simulink model "LAB7_OLD"  (R2021b)
settings: Solver=VariableStepDiscrete  StartTime=0.0  StopTime=100000  RelTol=1e-3  EnableMultiTasking=on
libraries: commchan3 x8, commdigbbndpm3 x8, commsink2 x8, commdigbbndam3 x8, commblkcod2 x8, commrandsrc3 x4
settings Model: Creator=The MathWorks, Inc.  LastModifiedBy=Argot
settings SolverCC: AlgebraicLoopSolver=TrustRegion
settings DataIOCC: LimitDataPoints=on  SaveFormat=Array  ReturnWorkspaceOutputs=off  SignalLoggingName=sigsOut
settings OptimizationCC: ExpressionDepthLimit=2147483647  InitFltsAndDblsToZero=on  LifeSpan=inf
settings DebuggingCC: SaveWithParameterizedLinksMsg=none  UnderspecifiedInitializationDetection=Classic  MergeDetectMultiDrivingBlocksExec=none  SignalResolutionControl=TryResolveAllWithWarning  MultiTaskDSMMsg=warning  MultiTaskCondExecSysMsg=none  FcnCallInpInsideContextMsg=warning  StateNameClashWarn=warning  SFUnexpectedBacktrackingDiag=warning  SFNoUnconditionalDefaultTransitionDiag=warning  SFExecutionAtInitializationDiag=none  SFMachineParentedDataDiag=warning  ArithmeticOperatorsInVariantConditions=warning
settings HardwareCC: ProdBitPerPointer=32  ProdBitPerSizeT=32  ProdBitPerPtrDiffT=32  ProdLargestAtomicFloat=None  ProdIntDivRoundTo=Undefined  ProdEndianess=Unspecified  ProdWordSize=32  ProdHWDeviceType=32-bit Generic  TargetUnknown=on
settings ModelReferenceCC: PropagateSignalLabelsOutOfModel=off
settings SFSimCC: SimUseLocalCustomCode=off  CustomCodeUndefinedFunction=UseInterfaceOnly
settings RTWCC: RTWUseLocalCustomCode=off
settings CodeAppCC: StateflowObjectComments=on
settings GRTTargetCC: TargetFcnLib=ansi_tfl_tmw.mat  TargetLangStandard=C89/C90 (ANSI)  CombineOutputUpdateFcns=off  GRTInterface=on
settings ConfigComp: CovMetricSettings=dw  CovSaveCumulativeToWorkspaceVar=on  CovSaveSingleToWorkspaceVar=on  CovExternalEMLEnable=off

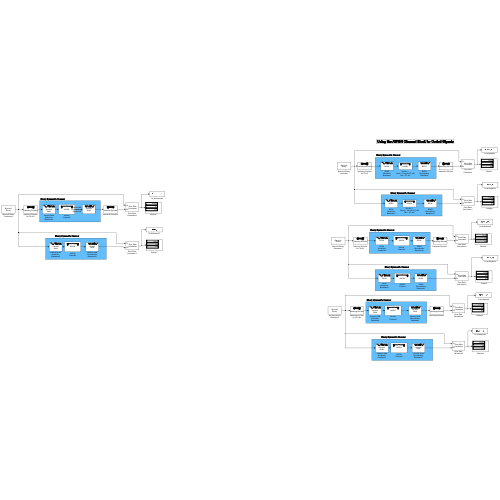
[thumbnail: Simulink's stored preview of the top-level diagram]
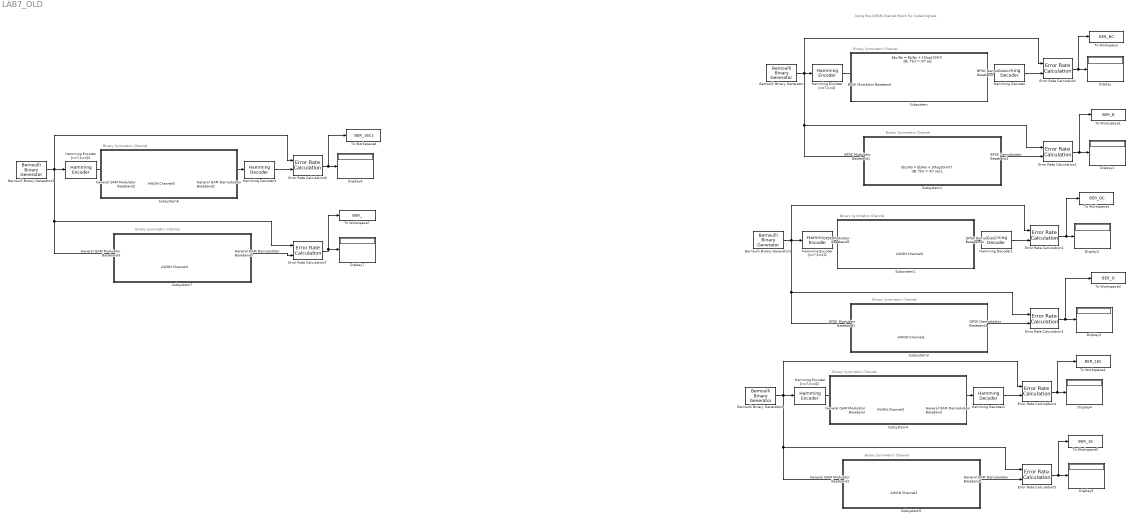
== system LAB7_OLD ==
  note: Binary Symmetric Channel
  note: Using the AWGN Channel Block for Coded Signals
  note: Binary Symmetric Channel
  note: Binary Symmetric Channel
  note: Binary Symmetric Channel
  note: Binary Symmetric Channel
  note: Binary Symmetric Channel
  note: Binary Symmetric Channel
  note: Binary Symmetric Channel
  AWGN Channel{1..3,6} (4 alike) : commchan3/AWGN Channel  InputProcessing=Columns as channels (frame based)  seed=67  noiseMode="Signal to noise ratio  (Eb/No)"  EbNodB=-40  EsNodB=10  SNRdB=10  bitsPerSym=1  Ps=1  Tsym=1  variance=1
  AWGN Channel4 : commchan3/AWGN Channel  InputProcessing=Columns as channels (frame based)  seed=67  noiseMode="Signal to noise ratio  (Eb/No)"  EbNodB=-2  EsNodB=10  SNRdB=10  bitsPerSym=1  Ps=1/1024  Tsym=1  variance=1
  AWGN Channel5 : commchan3/AWGN Channel  InputProcessing=Columns as channels (frame based)  seed=67  noiseMode="Signal to noise ratio  (Eb/No)"  EbNodB=-2  EsNodB=10  SNRdB=10  bitsPerSym=1  Ps=1/1024  Tsym=1  variance=1
  BPSK Demodulator Baseband : commdigbbndpm3/BPSK Demodulator Baseband  DecType=Hard decision  VarSource=Dialog  Variance=1  Ph=0  outDtype=double  derotateFactorWordLen=16  derotateFactorDataTypeStr=Inherit: Same word length as input  derotateFactorLastDataTypeStr=Inherit: Same word length as input
  BPSK Demodulator Baseband1 : commdigbbndpm3/BPSK Demodulator Baseband  DecType=Hard decision  VarSource=Dialog  Variance=1  Ph=0  outDtype=double  derotateFactorWordLen=16  derotateFactorDataTypeStr=Inherit: Same word length as input  derotateFactorLastDataTypeStr=Inherit: Same word length as input
  BPSK Modulator Baseband : commdigbbndpm3/BPSK Modulator Baseband  Ph=0  outDtype=double  outWordLen=16  outUDDataType=sfix(16)  outFracLenMode=Best precision  outFracLen=15  outDataTypeStr=double  outLastDataTypeStr=double
  BPSK Modulator Baseband1 : commdigbbndpm3/BPSK Modulator Baseband  Ph=0  outDtype=double  outWordLen=16  outUDDataType=sfix(16)  outFracLenMode=Best precision  outFracLen=15  outDataTypeStr=double  outLastDataTypeStr=double
  Bernoulli Binary Generator{,1..3} (4 alike) : commrandsrc3/Bernoulli Binary Generator  ProbabilityOfZero=0.5  SeedSource=Auto  Seed=0  SampleTime=1  SamplesPerFrame=4  OutputDataType=double  SimulateUsing=Interpreted execution
  Display{,1..7} (8 alike) : Display
  "Ebc/No = Eb/No + 10log10(4/7) dB, Tbit = 4/7 sec" : commchan3/AWGN Channel  InputProcessing=Columns as channels (frame based)  seed=67  noiseMode="Signal to noise ratio  (Eb/No)"  EbNodB=-40  EsNodB=6.75 + 10*log10(4/7)  SNRdB=10  bitsPerSym=1  Ps=1  Tsym=1  variance=1
  "Ebc/No = Eb/No + 10log10(4/7) dB, Tbit = 4/7 sec1" : commchan3/AWGN Channel  InputProcessing=Columns as channels (frame based)  seed=67  noiseMode="Signal to noise ratio  (Eb/No)"  EbNodB=-40  EsNodB=6.75 + 10*log10(4/7)  SNRdB=10  bitsPerSym=1  Ps=1  Tsym=1  variance=1
  Error Rate Calculation{,1..7} (8 alike) : commsink2/Error Rate Calculation  N=0  st_delay=0  cp_mode=Entire frame  subframe=[]  PMode=Port  WsName=ErrorVec  RsMode2=off  stop=on  numErr=200  maxBits=1e6
  General QAM Demodulator Baseband : commdigbbndam3/General QAM Demodulator Baseband  SigCon=[exp(2*pi*1i*[0:7]/8)]  OutType=Integer  DecType=Hard decision  VarSource=Dialog  Variance=1  outDtypeBit=Inherit via internal rule  outDtype=Inherit via internal rule  roundingMode=Floor  overflowMode=Wrap  OvFlMode=off  OvFlModeLastStrValue=off  sigConstWordLen=16  sigConstDataTypeStr=Inherit: Same word length as input  sigConstLastDataTypeStr=Inherit: Same word length as input  accum1WordLen=32  accum1FracLen=30  prodInWordLen=32  prodInFracLen=30  prodInDataTypeStr=Inherit: Same as accumulator 1  prodInLastDataTypeStr=Inherit: Same as accumulator 1  prodOutWordLen=32  prodOutFracLen=30  accum2WordLen=32  accum2FracLen=30  accum3WordLen=32  accum3FracLen=30  nsiWordLen=32  nsiFracLen=30  nsiDataTypeStr=Inherit: Same as accumulator 3  nsiLastDataTypeStr=Inherit: Same as accumulator 3  invn0WordLen=16  invn0FracLen=8  invn0DataTypeStr=Inherit: Same word length as input  invn0LastDataTypeStr=Inherit: Same word length as input  outputWordLen=32  outputFracLen=30
      settings: SourceProductBaseCode=CM
  General QAM Demodulator Baseband1 : commdigbbndam3/General QAM Demodulator Baseband  SigCon=[exp(2*pi*1i*[0:7]/8)]  OutType=Integer  DecType=Hard decision  VarSource=Dialog  Variance=1  outDtypeBit=Inherit via internal rule  outDtype=Inherit via internal rule  roundingMode=Floor  overflowMode=Wrap  OvFlMode=off  OvFlModeLastStrValue=off  sigConstWordLen=16  sigConstDataTypeStr=Inherit: Same word length as input  sigConstLastDataTypeStr=Inherit: Same word length as input  accum1WordLen=32  accum1FracLen=30  prodInWordLen=32  prodInFracLen=30  prodInDataTypeStr=Inherit: Same as accumulator 1  prodInLastDataTypeStr=Inherit: Same as accumulator 1  prodOutWordLen=32  prodOutFracLen=30  accum2WordLen=32  accum2FracLen=30  accum3WordLen=32  accum3FracLen=30  nsiWordLen=32  nsiFracLen=30  nsiDataTypeStr=Inherit: Same as accumulator 3  nsiLastDataTypeStr=Inherit: Same as accumulator 3  invn0WordLen=16  invn0FracLen=8  invn0DataTypeStr=Inherit: Same word length as input  invn0LastDataTypeStr=Inherit: Same word length as input  outputWordLen=32  outputFracLen=30
      settings: SourceProductBaseCode=CM
  General QAM Demodulator Baseband2 : commdigbbndam3/General QAM Demodulator Baseband  SigCon=[exp(2*pi*1i*[0:1023]/1024)]  OutType=Integer  DecType=Hard decision  VarSource=Dialog  Variance=1  outDtypeBit=Inherit via internal rule  outDtype=Inherit via internal rule  roundingMode=Floor  overflowMode=Wrap  OvFlMode=off  OvFlModeLastStrValue=off  sigConstWordLen=16  sigConstDataTypeStr=Inherit: Same word length as input  sigConstLastDataTypeStr=Inherit: Same word length as input  accum1WordLen=32  accum1FracLen=30  prodInWordLen=32  prodInFracLen=30  prodInDataTypeStr=Inherit: Same as accumulator 1  prodInLastDataTypeStr=Inherit: Same as accumulator 1  prodOutWordLen=32  prodOutFracLen=30  accum2WordLen=32  accum2FracLen=30  accum3WordLen=32  accum3FracLen=30  nsiWordLen=32  nsiFracLen=30  nsiDataTypeStr=Inherit: Same as accumulator 3  nsiLastDataTypeStr=Inherit: Same as accumulator 3  invn0WordLen=16  invn0FracLen=8  invn0DataTypeStr=Inherit: Same word length as input  invn0LastDataTypeStr=Inherit: Same word length as input  outputWordLen=32  outputFracLen=30
      settings: SourceProductBaseCode=CM
  General QAM Demodulator Baseband3 : commdigbbndam3/General QAM Demodulator Baseband  SigCon=[exp(2*pi*1i*[0:1023]/1024)]  OutType=Integer  DecType=Hard decision  VarSource=Dialog  Variance=1  outDtypeBit=Inherit via internal rule  outDtype=Inherit via internal rule  roundingMode=Floor  overflowMode=Wrap  OvFlMode=off  OvFlModeLastStrValue=off  sigConstWordLen=16  sigConstDataTypeStr=Inherit: Same word length as input  sigConstLastDataTypeStr=Inherit: Same word length as input  accum1WordLen=32  accum1FracLen=30  prodInWordLen=32  prodInFracLen=30  prodInDataTypeStr=Inherit: Same as accumulator 1  prodInLastDataTypeStr=Inherit: Same as accumulator 1  prodOutWordLen=32  prodOutFracLen=30  accum2WordLen=32  accum2FracLen=30  accum3WordLen=32  accum3FracLen=30  nsiWordLen=32  nsiFracLen=30  nsiDataTypeStr=Inherit: Same as accumulator 3  nsiLastDataTypeStr=Inherit: Same as accumulator 3  invn0WordLen=16  invn0FracLen=8  invn0DataTypeStr=Inherit: Same word length as input  invn0LastDataTypeStr=Inherit: Same word length as input  outputWordLen=32  outputFracLen=30
      settings: SourceProductBaseCode=CM
  General QAM Modulator Baseband : commdigbbndam3/General QAM Modulator Baseband  SigCon=[exp(2*pi*1i*[0:7]/8)]  outDtype=double  outWordLen=16  outUDDataType=sfix(16)  outFracLenMode=Best precision  outFracLen=15  outDataTypeStr=double  outLastDataTypeStr=double
      settings: SourceProductBaseCode=CM
  General QAM Modulator Baseband1 : commdigbbndam3/General QAM Modulator Baseband  SigCon=[exp(2*pi*1i*[0:7]/8)]  outDtype=double  outWordLen=16  outUDDataType=sfix(16)  outFracLenMode=Best precision  outFracLen=15  outDataTypeStr=double  outLastDataTypeStr=double
      settings: SourceProductBaseCode=CM
  General QAM Modulator Baseband2 : commdigbbndam3/General QAM Modulator Baseband  SigCon=[exp(2*pi*1i*[0:1023]/1024)]  outDtype=double  outWordLen=16  outUDDataType=sfix(16)  outFracLenMode=Best precision  outFracLen=15  outDataTypeStr=double  outLastDataTypeStr=double
      settings: SourceProductBaseCode=CM
  General QAM Modulator Baseband3 : commdigbbndam3/General QAM Modulator Baseband  SigCon=[exp(2*pi*1i*[0:1023]/1024)]  outDtype=double  outWordLen=16  outUDDataType=sfix(16)  outFracLenMode=Best precision  outFracLen=15  outDataTypeStr=double  outLastDataTypeStr=double
      settings: SourceProductBaseCode=CM
  Hamming Decoder{,1..3} (4 alike) : commblkcod2/Hamming Decoder  n=7  k=4
      settings: SourceProductBaseCode=CM
  Hamming Encoder [n=7,k=4]{,1..3} (4 alike) : commblkcod2/Hamming Encoder  n=7  k=4
      settings: SourceProductBaseCode=CM
  QPSK Demodulator Baseband1 : commdigbbndpm3/QPSK Demodulator Baseband  OutType=Integer  DecType=Hard decision  VarSource=Dialog  Variance=1  Dec=Gray  Ph=pi/4  outDtype1=Inherit via internal rule  outDtype2=Inherit via internal rule  derotateFactorWordLen=16  derotateFactorDataTypeStr=Inherit: Same word length as input  derotateFactorLastDataTypeStr=Inherit: Same word length as input
  QPSK Demodulator Baseband4 : commdigbbndpm3/QPSK Demodulator Baseband  OutType=Integer  DecType=Hard decision  VarSource=Dialog  Variance=1  Dec=Gray  Ph=pi/4  outDtype1=Inherit via internal rule  outDtype2=Inherit via internal rule  derotateFactorWordLen=16  derotateFactorDataTypeStr=Inherit: Same word length as input  derotateFactorLastDataTypeStr=Inherit: Same word length as input
  QPSK Modulator Baseband1 : commdigbbndpm3/QPSK Modulator Baseband  InType=Integer  Enc=Gray  Ph=pi/4  outDtype=double  outWordLen=16  outUDDataType=sfix(16)  outFracLenMode=Best precision  outFracLen=15  outDataTypeStr=double  outLastDataTypeStr=double
  QPSK Modulator Baseband5 : commdigbbndpm3/QPSK Modulator Baseband  InType=Integer  Enc=Gray  Ph=pi/4  outDtype=double  outWordLen=16  outUDDataType=sfix(16)  outFracLenMode=Best precision  outFracLen=15  outDataTypeStr=double  outLastDataTypeStr=double
  Subsystem : Subsystem
      mask Display: disp('')
  Subsystem1 : Subsystem
      mask Display: disp('')
  Subsystem2 : Subsystem
      mask Display: disp('')
  Subsystem3 : Subsystem
      mask Display: disp('')
  Subsystem4 : Subsystem
      mask Display: disp('')
  Subsystem5 : Subsystem
      mask Display: disp('')
  Subsystem6 : Subsystem
      mask Display: disp('')
  Subsystem7 : Subsystem
      mask Display: disp('')
  To Workspace : ToWorkspace  VariableName=BER_BC  SaveFormat=Timeseries  SampleTime=-1
  To Workspace1 : ToWorkspace  VariableName=BER_B  SaveFormat=Timeseries  SampleTime=-1
  To Workspace2 : ToWorkspace  VariableName=BER_QC  SaveFormat=Timeseries  SampleTime=-1
  To Workspace3 : ToWorkspace  VariableName=BER_Q  SaveFormat=Timeseries  SampleTime=-1
  To Workspace4 : ToWorkspace  VariableName=BER_16C  SaveFormat=Timeseries  SampleTime=-1
  To Workspace5 : ToWorkspace  VariableName=BER_16  SaveFormat=Timeseries  SampleTime=-1
  To Workspace6 : ToWorkspace  VariableName=BER_16C1  SaveFormat=Timeseries  SampleTime=-1
  To Workspace7 : ToWorkspace  VariableName=BER_  SaveFormat=Timeseries  SampleTime=-1
  wires:
  BPSK Modulator Baseband/1 -> "Ebc/No = Eb/No + 10log10(4/7) dB, Tbit = 4/7 sec"/1
  "Ebc/No = Eb/No + 10log10(4/7) dB, Tbit = 4/7 sec"/1 -> BPSK Demodulator Baseband/1
  Error Rate Calculation/1 -> To Workspace/1, Display/1
  Bernoulli Binary Generator/1 -> Hamming Encoder [n=7,k=4]/1, Error Rate Calculation/1, BPSK Modulator Baseband1/1, Error Rate Calculation1/1
  Hamming Encoder [n=7,k=4]/1 -> BPSK Modulator Baseband/1
  BPSK Demodulator Baseband/1 -> Hamming Decoder/1
  Hamming Decoder/1 -> Error Rate Calculation/2
  BPSK Demodulator Baseband1/1 -> Error Rate Calculation1/2
  Error Rate Calculation1/1 -> To Workspace1/1, Display1/1
  "Ebc/No = Eb/No + 10log10(4/7) dB, Tbit = 4/7 sec1"/1 -> BPSK Demodulator Baseband1/1
  BPSK Modulator Baseband1/1 -> "Ebc/No = Eb/No + 10log10(4/7) dB, Tbit = 4/7 sec1"/1
  Error Rate Calculation3/1 -> To Workspace3/1, Display3/1
  Bernoulli Binary Generator1/1 -> Hamming Encoder [n=7,k=4]1/1, Error Rate Calculation2/1, QPSK Modulator Baseband1/1, Error Rate Calculation3/1
  Error Rate Calculation2/1 -> To Workspace2/1, Display2/1
  Hamming Decoder1/1 -> Error Rate Calculation2/2
  Hamming Encoder [n=7,k=4]1/1 -> QPSK Modulator Baseband5/1
  QPSK Modulator Baseband5/1 -> AWGN Channel6/1
  AWGN Channel6/1 -> QPSK Demodulator Baseband4/1
  QPSK Demodulator Baseband4/1 -> Hamming Decoder1/1
  QPSK Modulator Baseband1/1 -> AWGN Channel1/1
  AWGN Channel1/1 -> QPSK Demodulator Baseband1/1
  QPSK Demodulator Baseband1/1 -> Error Rate Calculation3/2
  General QAM Demodulator Baseband1/1 -> Error Rate Calculation5/2
  AWGN Channel2/1 -> General QAM Demodulator Baseband1/1
  General QAM Modulator Baseband1/1 -> AWGN Channel2/1
  Hamming Decoder2/1 -> Error Rate Calculation4/2
  Error Rate Calculation4/1 -> To Workspace4/1, Display4/1
  Bernoulli Binary Generator2/1 -> General QAM Modulator Baseband1/1, Error Rate Calculation5/1, Error Rate Calculation4/1, Hamming Encoder [n=7,k=4]2/1
  Error Rate Calculation5/1 -> To Workspace5/1, Display5/1
  Hamming Encoder [n=7,k=4]2/1 -> General QAM Modulator Baseband/1
  General QAM Modulator Baseband/1 -> AWGN Channel3/1
  AWGN Channel3/1 -> General QAM Demodulator Baseband/1
  General QAM Demodulator Baseband/1 -> Hamming Decoder2/1
  Error Rate Calculation7/1 -> To Workspace7/1, Display7/1
  General QAM Demodulator Baseband2/1 -> Hamming Decoder3/1
  AWGN Channel5/1 -> General QAM Demodulator Baseband2/1
  General QAM Modulator Baseband2/1 -> AWGN Channel5/1
  Hamming Decoder3/1 -> Error Rate Calculation6/2
  Hamming Encoder [n=7,k=4]3/1 -> General QAM Modulator Baseband2/1
  Bernoulli Binary Generator3/1 -> General QAM Modulator Baseband3/1, Error Rate Calculation7/1, Error Rate Calculation6/1, Hamming Encoder [n=7,k=4]3/1
  General QAM Modulator Baseband3/1 -> AWGN Channel4/1
  General QAM Demodulator Baseband3/1 -> Error Rate Calculation7/2
  Error Rate Calculation6/1 -> To Workspace6/1, Display6/1
  AWGN Channel4/1 -> General QAM Demodulator Baseband3/1

== system LAB7_OLD/Subsystem ==

== system LAB7_OLD/Subsystem1 ==

== system LAB7_OLD/Subsystem2 ==

== system LAB7_OLD/Subsystem3 ==

== system LAB7_OLD/Subsystem4 ==

== system LAB7_OLD/Subsystem5 ==

== system LAB7_OLD/Subsystem6 ==

== system LAB7_OLD/Subsystem7 ==
